simulink model "six_rod_tensegrity_model_2021a"  (R2021a)
settings: Solver=ode45  StartTime=0  StopTime=Inf  RelTol=1e-1
values from neighbouring files (symbols this model uses):
  grivity_z = -9.80665    [code_for_6_rods_tensegrity.m]
  i = 19    [drive_params.m]
  Jsum = Jd + Jp + Jnagr    (= 9.27e-08)    [drive_params.m]
  km = 9.32 / 1000    (= 0.00932)    [drive_params.m]
  kpdr = 0.81    [drive_params.m]
  kw = 60 / (2*pi * 1020)    (= 0.00936205547599)    [drive_params.m]
  L = 0.14 / 1000    (= 0.00014)    [drive_params.m]
  load_mass = 0.5    [code_for_6_rods_tensegrity.m]
  plane_offset = -(rod_length/2 + 0.032 + rod_radius)    [code_for_6_rods_tensegrity.m]
  R = 5.3    [drive_params.m]
  rod_end_drive_offset = spool_active_length    (= 0.015)    [code_for_6_rods_tensegrity.m]
  rod_end_mass = 0.05    [code_for_6_rods_tensegrity.m]
  rod_end_mass_with_drive = 0.2    [code_for_6_rods_tensegrity.m]
  rod_mass = 0.028    [code_for_6_rods_tensegrity.m]
  rod_mass_with_drive = 0.038    [code_for_6_rods_tensegrity.m]
  rod_radius = 0.004    [code_for_6_rods_tensegrity.m]
undefined symbols (not defined in the file or in its folder): Left_end_cap_1_1, Left_end_cap_2_3, Left_end_cap_3_5, Left_end_cap_4_7, Left_end_cap_5_9, Left_end_cap_6_11, Right_end_cap_1_2, Right_end_cap_2_4, Right_end_cap_3_6, Right_end_cap_4_8, Right_end_cap_5_10, Right_end_cap_6_12, Rod_center_1, Rod_center_2, Rod_center_3, Rod_center_4, Rod_center_5, Rod_center_6, sigbuilder_block, X, Y, Z
libraries: sm_lib x403, nesl_utility x73
(part 1 of 5)
settings Model: SimulationMode=accelerator  Creator=skept  LastModifiedBy=Alexander
settings SolverCC: ZeroCrossAlgorithm=Adaptive  AlgebraicLoopSolver=TrustRegion  MinimalZcImpactIntegration=on
settings DataIOCC: LimitDataPoints=on  ReturnWorkspaceOutputs=off
settings OptimizationCC: LifeSpan=Inf
settings DebuggingCC: ReadBeforeWriteMsg=DisableAll  WriteAfterWriteMsg=DisableAll  WriteAfterReadMsg=DisableAll  IgnoredZcDiagnostic=none  MultiTaskDSMMsg=none  SFMachineParentedDataDiag=warning  ArithmeticOperatorsInVariantConditions=warning
settings ModelReferenceCC: UpdateModelReferenceTargets=IfOutOfDate
settings SFSimCC: CustomCodeUndefinedFunction=UseInterfaceOnly  SimTargetLang=C++
settings ExplorerConfigSet: InternalSimMechanicsExplorerSettings="<ExplorerConfiguration><canonicalview>default</canonicalview><AnimationSetting><BasePlaybackSpeed>1.0</BasePlaybackSpeed><PlaybackSpeedFactor>1.0</PlaybackSpeedFactor></AnimationSetting><TilePanel><TileInfo><Tiles Columns=\"2\" Count=\"2\" Rows=\"1\"><Column Weight=\"0.4996\"/><Column Weight=\"0.5004\"/><Row Weight=\"1\"/><Tile Height=\"1\" Width=\"1\" X=\"0\" Y=\"0\"/><Tile Height=\"1\" Width=\"1\" X=\"1\" Y=\"0\"/></Tiles></TileInfo><SceneInfo><SceneViewer><BGColor><R>0.60000002384185791</R><G>0.60000002384185791</G><B>0.60000002384185791</B></BGColor><Camera><DoPerspective>off</DoPerspective><Position><X>4.6237270475932446</X><Y>-3.24046644242923998</Y><Z>4.39238714743132519</Z></Position><Center><X>-0.0432625823170843388</X><Y>0.165607191250739916</Y><Z>-0.253002280802875512</Z></Center><Up><X>-0.498867944911503491</X><Y>0.379278649695632186</Y><Z>0.779280744933962821</Z></Up><ViewLimDist>1</ViewLimDist><YLim>1.22665931905449344</YLim><XLim>0.999371665877494042</XLim></Camera></SceneViewer><SceneViewer><BGColor><R>0.60000002384185791</R><G>0.60000002384185791</G><B>0.60000002384185791</B></BGColor><Camera><DoPerspective>off</DoPerspective><Position><X>0.00285027965081703291</X><Y>-7.09077849007995908</Y><Z>0.0787782984999531449</Z></Position><Center><X>0.00285027965081703291</X><Y>1.92077906472493121e-07</Y><Z>0.0787782984999531449</Z></Center><Up><X>0</X><Y>-0</Y><Z>1</Z></Up><ViewLimDist>1</ViewLimDist><YLim>0.451172617625770545</YLim><XLim>0.368213013253280874</XLim></Camera></SceneViewer></SceneInfo></TilePanel><MechEditorPanel><Cameras/><GfxPanelCameraMap/><VideoCreator><PlaybackSpeedRatio>1.0</PlaybackSpeedRatio><FrameRate>60</FrameRate><VideoFormat>MPEG-4</VideoFormat><FrameSize>[1920 1080]</FrameSize></VideoCreator></MechEditorPanel></ExplorerConfiguration>"

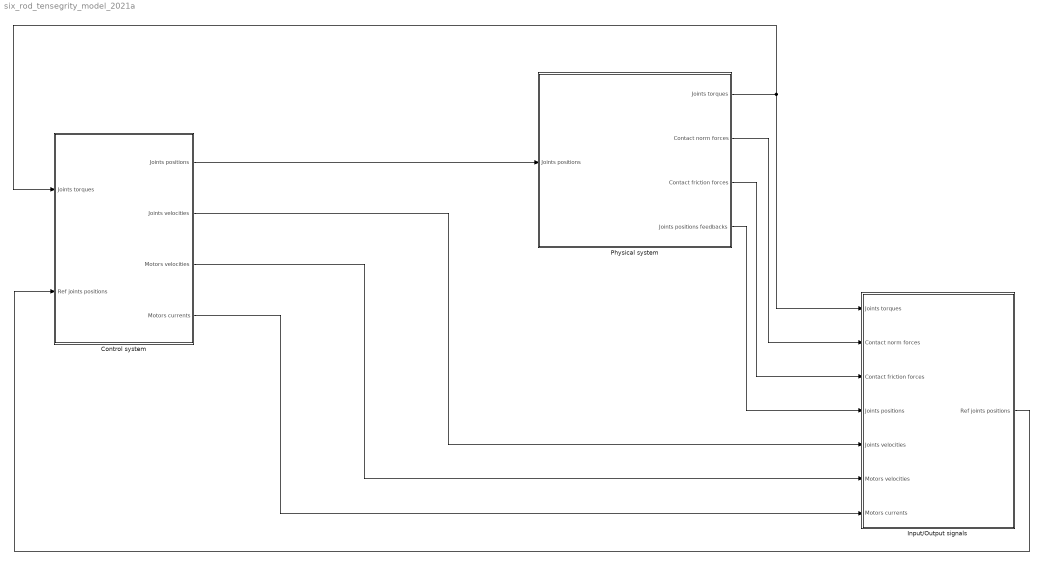
== system six_rod_tensegrity_model_2021a ==
  Control system : Subsystem
  Input/Output signals : Subsystem
  Physical system : Subsystem
      mask Display: image('$imagefile'); % Use "Edit Image" on toolstrip to change.
  wires:
  Control system/1(Joints positions) -> Physical system/1(Joints positions)
  Physical system/1(Joints torques) -> Input/Output signals/1(Joints torques), Control system/1(Joints torques)
  Control system/2(Joints velocities) -> Input/Output signals/5(Joints velocities)
  Control system/3(Motors velocities) -> Input/Output signals/6(Motors velocities)
  Control system/4(Motors currents) -> Input/Output signals/7(Motors currents)
  Input/Output signals/1(Ref joints positions) -> Control system/2(Ref joints positions)
  Physical system/2(Contact norm forces) -> Input/Output signals/2(Contact norm forces)
  Physical system/3(Contact friction forces) -> Input/Output signals/3(Contact friction forces)
  Physical system/4(Joints positions feedbacks) -> Input/Output signals/4(Joints positions)

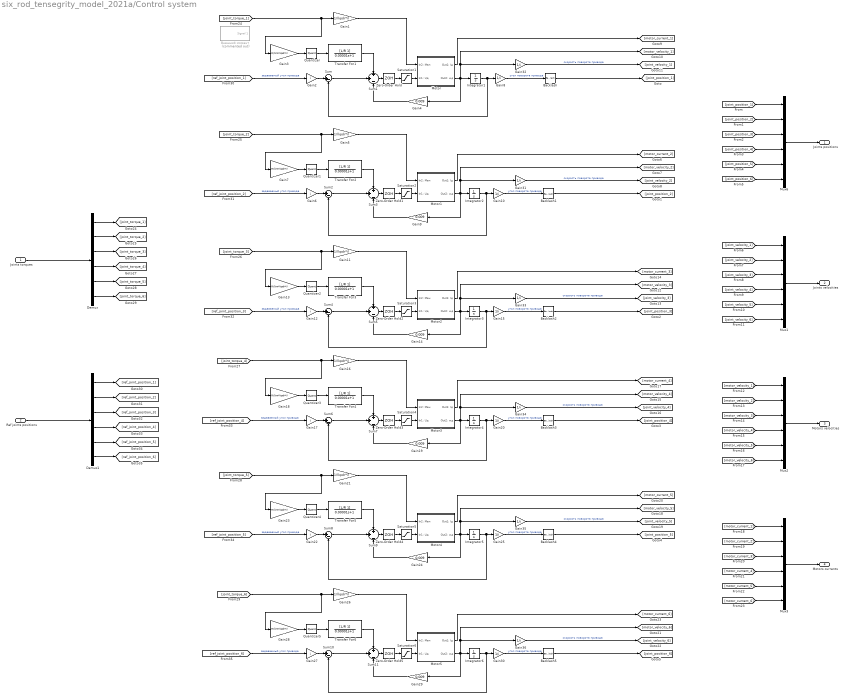
== system six_rod_tensegrity_model_2021a/Control system ==
  Joints torques : Inport
  Ref joints positions : Inport  Port=2
  Backlash{,1..5} (6 alike) : Backlash  BacklashWidth=0.0279
  Demux : Demux  Outputs=6
  Demux1 : Demux  Outputs=6
  Gain{1,5,11,16,21,26} (6 alike) : Gain  Gain=1/(kpdr*i)
  Gain{8,10,15,20,25,30..36} (12 alike) : Gain  Gain=1/i
  Gain{2,6,12,17,22,27} (6 alike) : Gain  Gain=i
  Gain{3,7,13,18,23,28} (6 alike) : Gain  Gain=R/(km*kpdr*i)
  Gain{4,9,14,19,24,29} (6 alike) : Gain  Gain=0.009
  Integrator{1..6} (6 alike) : Integrator
  Motor : Subsystem
  Motor1 : Subsystem
  Motor2 : Subsystem
  Motor3 : Subsystem
  Motor4 : Subsystem
  Motor5 : Subsystem
  Mux{1..3,6} (4 alike) : Mux  Inputs=6
  Quantizer{,1..5} (6 alike) : Quantizer  QuantizationInterval=0.00488
  Saturation{1..6} (6 alike) : Saturate  UpperLimit=10.8  LowerLimit=-10.8
  Sum{,2,4,6,8,10} (6 alike) : Sum  Inputs=|+-
  Sum{1,3,5,7,9,11} (6 alike) : Sum  Inputs=+|+|-
  Transfer Fcn{1..6} (6 alike) : TransferFcn  Numerator=[L/R 1]  Denominator=[0.00001 1]
  Zero-Order Hold{,1..5} (6 alike) : ZeroOrderHold  SampleTime=0.005
  Внешний момент : Subsystem  Tag=STV Subsys  Commented=on  LoadFcn=sigbuilder_block('load');  StartFcn=sigbuilder_block('start');  StopFcn=sigbuilder_block('stop');  ClipboardFcn=sigbuilder_block('clipboard');  mask(Sigbuilder block){tuvar=[0:10]}
      mask help: Simulink:masks:SigbuilderBlock_MD
      mask init:
      | if ~strcmp(get_param(bdroot(gcbh),'SimulationStatus'),'stopped') tuvar = sigbuilder_block('maskInit'); end
      settings: CopyFcn=sigbuilder_block('copy');  DeleteFcn=sigbuilder_block('delete');  ModelCloseFcn=sigbuilder_block('modelClose');  PreSaveFcn=sigbuilder_block('preSave');  PauseFcn=sigbuilder_block('pause');  ContinueFcn=sigbuilder_block('continue');  NameChangeFcn=sigbuilder_block('namechange');  OpenFcn=sigbuilder_block('open',[512.25 154.5 550.5 399.75 ]);  CloseFcn=sigbuilder_block('close');
      mask Display: plot(0, 0, 100, 100,[2, 2, 32, 32, 2], [68, 8, 8, 68, 68],[32, 2], [38, 38], [32, 19, 2],[53, 60, 44], [32, 17, 17, 2],[16, 16, 31, 31]);txt = getActiveGroup(gcbh);text(2, 100, txt,'verticalAlignment', 'top');
  Joints positions : Outport
  Joints velocities : Outport  Port=2
  Motors velocities : Outport  Port=3
  Motors currents : Outport  Port=4
  wires:
  Gain1/1 -> Motor/1(In2: Mвн)
  Backlash/1 -> [joint_position_1]
  [joint_torque_1] -> Gain1/1, Gain3/1
  Quantizer/1 -> Transfer Fcn1/1
  Gain4/1 -> Sum1/3
  Gain2/1 -> Sum/1
  Sum/1 -> Sum1/2
  Transfer Fcn1/1 -> Sum1/1
  Gain3/1 -> Quantizer/1
  [ref_joint_position_1] -> Gain2/1  "задаваемый угол привода"
  Integrator1/1 -> Gain8/1, Sum/2
  Zero-Order Hold/1 -> Saturation1/1
  Saturation1/1 -> Motor/2(In1: Uд)
  Sum1/1 -> Zero-Order Hold/1
  Motor/2(Out2: wд) -> [motor_velocity_1], Gain32/1, Integrator1/1, Gain4/1
  Gain8/1 -> Backlash/1  "угол поворота привода"
  Motor1/2(Out2: wд) -> Gain31/1, [motor_velocity_2], Gain9/1, Integrator2/1
  Integrator2/1 -> Gain10/1, Sum2/2
  Zero-Order Hold1/1 -> Saturation2/1
  Gain10/1 -> Backlash1/1  "угол поворота привода"
  Sum3/1 -> Zero-Order Hold1/1
  Transfer Fcn2/1 -> Sum3/1
  Gain9/1 -> Sum3/3
  [ref_joint_position_2] -> Gain6/1  "задаваемый угол привода"
  Gain7/1 -> Quantizer1/1
  Sum2/1 -> Sum3/2
  [joint_torque_2] -> Gain5/1, Gain7/1
  Quantizer1/1 -> Transfer Fcn2/1
  Gain6/1 -> Sum2/1
  Backlash1/1 -> [joint_position_2]
  Gain5/1 -> Motor1/1(In2: Mвн)
  Saturation2/1 -> Motor1/2(In1: Uд)
  Motor2/2(Out2: wд) -> Gain33/1, [motor_velocity_3], Gain14/1, Integrator3/1
  Integrator3/1 -> Gain15/1, Sum4/2
  Zero-Order Hold2/1 -> Saturation3/1
  Gain15/1 -> Backlash2/1  "угол поворота привода"
  Sum5/1 -> Zero-Order Hold2/1
  Transfer Fcn3/1 -> Sum5/1
  Gain14/1 -> Sum5/3
  [ref_joint_position_3] -> Gain12/1  "задаваемый угол привода"
  Gain13/1 -> Quantizer2/1
  Sum4/1 -> Sum5/2
  [joint_torque_3] -> Gain11/1, Gain13/1
  Quantizer2/1 -> Transfer Fcn3/1
  Gain12/1 -> Sum4/1
  Backlash2/1 -> [joint_position_3]
  Gain11/1 -> Motor2/1(In2: Mвн)
  Saturation3/1 -> Motor2/2(In1: Uд)
  Motor3/2(Out2: wд) -> [motor_velocity_4], Gain34/1, Integrator4/1, Gain19/1
  Integrator4/1 -> Gain20/1, Sum6/2
  Zero-Order Hold3/1 -> Saturation4/1
  Gain20/1 -> Backlash3/1  "угол поворота привода"
  Sum7/1 -> Zero-Order Hold3/1
  Transfer Fcn4/1 -> Sum7/1
  Gain19/1 -> Sum7/3
  [ref_joint_position_4] -> Gain17/1  "задаваемый угол привода"
  Gain18/1 -> Quantizer3/1
  Sum6/1 -> Sum7/2
  [joint_torque_4] -> Gain16/1, Gain18/1
  Quantizer3/1 -> Transfer Fcn4/1
  Gain17/1 -> Sum6/1
  Backlash3/1 -> [joint_position_4]
  Gain16/1 -> Motor3/1(In2: Mвн)
  Saturation4/1 -> Motor3/2(In1: Uд)
  Integrator5/1 -> Gain25/1, Sum8/2
  Zero-Order Hold4/1 -> Saturation5/1
  Gain25/1 -> Backlash4/1  "угол поворота привода"
  Sum9/1 -> Zero-Order Hold4/1
  Transfer Fcn5/1 -> Sum9/1
  Gain24/1 -> Sum9/3
  [ref_joint_position_5] -> Gain22/1  "задаваемый угол привода"
  Gain23/1 -> Quantizer4/1
  Sum8/1 -> Sum9/2
  [joint_torque_5] -> Gain21/1, Gain23/1
  Quantizer4/1 -> Transfer Fcn5/1
  Gain22/1 -> Sum8/1
  Backlash4/1 -> [joint_position_5]
  Gain21/1 -> Motor4/1(In2: Mвн)
  Saturation5/1 -> Motor4/2(In1: Uд)
  Motor5/2(Out2: wд) -> [motor_velocity_6], Gain36/1, Integrator6/1, Gain29/1
  Integrator6/1 -> Gain30/1, Sum10/2
  Zero-Order Hold5/1 -> Saturation6/1
  Gain30/1 -> Backlash5/1  "угол поворота привода"
  Sum11/1 -> Zero-Order Hold5/1
  Transfer Fcn6/1 -> Sum11/1
  Gain29/1 -> Sum11/3
  [ref_joint_position_6] -> Gain27/1  "задаваемый угол привода"
  Gain28/1 -> Quantizer5/1
  Sum10/1 -> Sum11/2
  [joint_torque_6] -> Gain26/1, Gain28/1
  Quantizer5/1 -> Transfer Fcn6/1
  Gain27/1 -> Sum10/1
  Backlash5/1 -> [joint_position_6]
  Gain26/1 -> Motor5/1(In2: Mвн)
  Saturation6/1 -> Motor5/2(In1: Uд)
  Mux6/1 -> Joints positions/1
  [joint_position_6] -> Mux6/6
  [joint_position_5] -> Mux6/5
  [joint_position_4] -> Mux6/4
  [joint_position_3] -> Mux6/3
  [joint_position_2] -> Mux6/2
  [joint_position_1] -> Mux6/1
  Motor1/1(Out1: Iд) -> [motor_current_2]
  Gain31/1 -> [joint_velocity_2]  "скорость поворота привода"
  Gain32/1 -> [joint_velocity_1]  "скорость поворота привода"
  Motor/1(Out1: Iд) -> [motor_current_1]
  Gain33/1 -> [joint_velocity_3]  "скорость поворота привода"
  Motor2/1(Out1: Iд) -> [motor_current_3]
  Gain34/1 -> [joint_velocity_4]  "скорость поворота привода"
  Motor3/1(Out1: Iд) -> [motor_current_4]
  Gain35/1 -> [joint_velocity_5]  "скорость поворота привода"
  Motor4/2(Out2: wд) -> Gain24/1, Gain35/1, [motor_velocity_5], Integrator5/1
  Motor4/1(Out1: Iд) -> [motor_current_5]
  Gain36/1 -> [joint_velocity_6]  "скорость поворота привода"
  Motor5/1(Out1: Iд) -> [motor_current_6]
  [joint_velocity_2] -> Mux1/2
  [joint_velocity_1] -> Mux1/1
  [joint_velocity_3] -> Mux1/3
  Mux1/1 -> Joints velocities/1
  [joint_velocity_4] -> Mux1/4
  [joint_velocity_5] -> Mux1/5
  [joint_velocity_6] -> Mux1/6
  [motor_velocity_2] -> Mux2/2
  [motor_velocity_1] -> Mux2/1
  [motor_velocity_3] -> Mux2/3
  Mux2/1 -> Motors velocities/1
  [motor_velocity_4] -> Mux2/4
  [motor_velocity_5] -> Mux2/5
  [motor_velocity_6] -> Mux2/6
  [motor_current_2] -> Mux3/2
  [motor_current_1] -> Mux3/1
  [motor_current_3] -> Mux3/3
  Mux3/1 -> Motors currents/1
  [motor_current_4] -> Mux3/4
  [motor_current_5] -> Mux3/5
  [motor_current_6] -> Mux3/6
  Demux/1 -> [joint_torque_1]
  Demux/2 -> [joint_torque_2]
  Demux/3 -> [joint_torque_3]
  Demux/6 -> [joint_torque_6]
  Joints torques/1 -> Demux/1
  Demux/4 -> [joint_torque_4]
  Demux/5 -> [joint_torque_5]
  Demux1/6 -> [ref_joint_position_6]
  Demux1/3 -> [ref_joint_position_3]
  Demux1/1 -> [ref_joint_position_1]
  Demux1/2 -> [ref_joint_position_2]
  Ref joints positions/1 -> Demux1/1
  Demux1/4 -> [ref_joint_position_4]
  Demux1/5 -> [ref_joint_position_5]

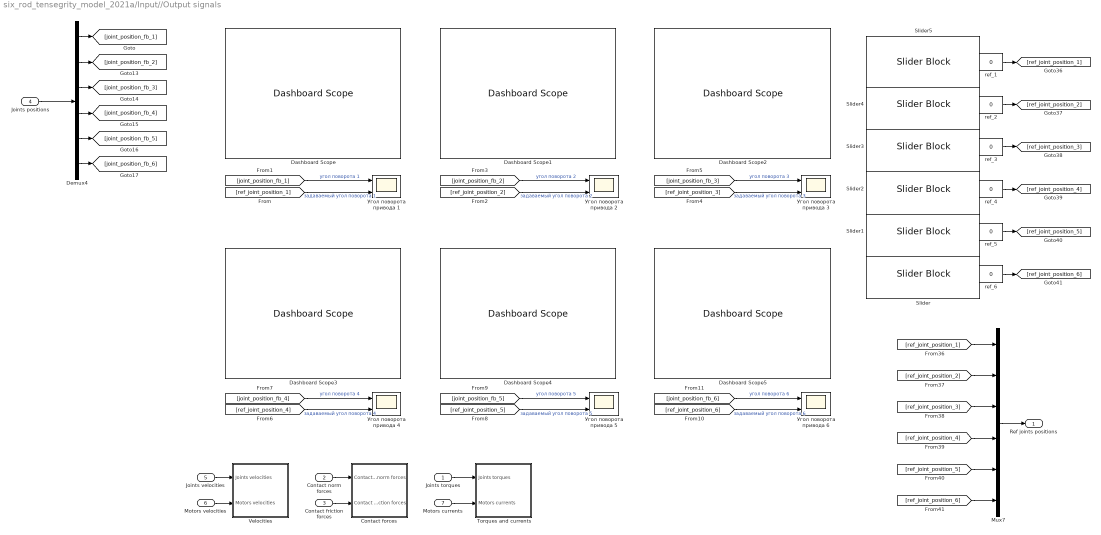
== system six_rod_tensegrity_model_2021a/Input//Output signals ==
  Joints torques : Inport
  Contact norm forces : Inport  Port=2
  Contact friction forces : Inport  Port=3
  Joints positions : Inport  Port=4
  Joints velocities : Inport  Port=5
  Motors velocities : Inport  Port=6
  Motors currents : Inport  Port=7
  Contact forces : Subsystem
  Dashboard Scope{,1..5} (6 alike) : DashboardScope
  Demux4 : Demux  Outputs=6
  Mux7 : Mux  Inputs=6
  Slider{,1..5} (6 alike) : SliderBlock  ScaleMax=200
  Torques and currents : Subsystem
  Velocities : Subsystem
  ref_{1..6} (6 alike) : Constant  Value=0
  Угол поворота привода {1..6} (6 alike) : Scope  NumInputPorts=2
  Ref joints positions : Outport
  wires:
  Demux4/1 -> [joint_position_fb_1]
  Demux4/2 -> [joint_position_fb_2]
  Demux4/3 -> [joint_position_fb_3]
  Demux4/6 -> [joint_position_fb_6]
  Joints positions/1 -> Demux4/1
  Demux4/4 -> [joint_position_fb_4]
  Demux4/5 -> [joint_position_fb_5]
  [ref_joint_position_1] -> Угол поворота привода 1/2  "задаваемый угол поворота 1"
  [joint_position_fb_1] -> Угол поворота привода 1/1  "угол поворота 1"
  [joint_position_fb_2] -> Угол поворота привода 2/1  "угол поворота 2"
  [ref_joint_position_2] -> Угол поворота привода 2/2  "задаваемый угол поворота 2"
  [joint_position_fb_3] -> Угол поворота привода 3/1  "угол поворота 3"
  [ref_joint_position_3] -> Угол поворота привода 3/2  "задаваемый угол поворота 3"
  [joint_position_fb_4] -> Угол поворота привода 4/1  "угол поворота 4"
  [ref_joint_position_4] -> Угол поворота привода 4/2  "задаваемый угол поворота 4"
  [joint_position_fb_5] -> Угол поворота привода 5/1  "угол поворота 5"
  [ref_joint_position_5] -> Угол поворота привода 5/2  "задаваемый угол поворота 5"
  [joint_position_fb_6] -> Угол поворота привода 6/1  "угол поворота 6"
  [ref_joint_position_6] -> Угол поворота привода 6/2  "задаваемый угол поворота 6"
  ref_5/1 -> [ref_joint_position_5]
  ref_2/1 -> [ref_joint_position_2]
  ref_6/1 -> [ref_joint_position_6]
  ref_4/1 -> [ref_joint_position_4]
  ref_1/1 -> [ref_joint_position_1]
  [ref_joint_position_1] -> Mux7/1
  [ref_joint_position_5] -> Mux7/5
  Mux7/1 -> Ref joints positions/1
  [ref_joint_position_3] -> Mux7/3
  [ref_joint_position_6] -> Mux7/6
  [ref_joint_position_4] -> Mux7/4
  [ref_joint_position_2] -> Mux7/2
  ref_3/1 -> [ref_joint_position_3]
  Contact norm forces/1 -> Contact forces/1(Contact norm forces)
  Contact friction forces/1 -> Contact forces/2(Contact friction forces)
  Joints velocities/1 -> Velocities/1(Joints velocities)
  Motors velocities/1 -> Velocities/2(Motors velocities)
  Joints torques/1 -> Torques and currents/1(Joints torques)
  Motors currents/1 -> Torques and currents/2(Motors currents)

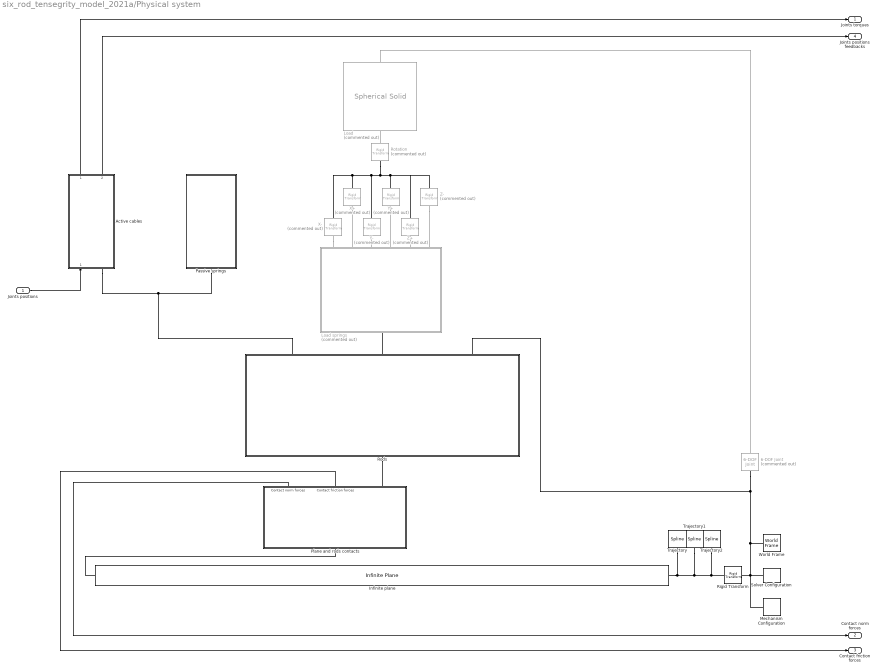
== system six_rod_tensegrity_model_2021a/Physical system ==
  Joints positions : Inport
  6-DOF Joint : sm_lib/Joints/6-DOF Joint  Commented=on  JointMode=Normal  SenseConstraintForce=off  SenseConstraintForceX=off  SenseConstraintForceY=off  SenseConstraintForceZ=off  SenseConstraintTorque=off  SenseConstraintTorqueX=off  SenseConstraintTorqueY=off  SenseConstraintTorqueZ=off  SenseTotalForce=off  SenseTotalForceX=off  SenseTotalForceY=off  SenseTotalForceZ=off  SenseTotalTorque=off  SenseTotalTorqueX=off  SenseTotalTorqueY=off  SenseTotalTorqueZ=off  CompositeWrenchDir=FollowerOnBase  CompositeWrenchFrame=BaseFrame  PxEquilibriumPosition=0  PxEquilibriumPositionUnits=m  PxSpringStiffness=0  PxSpringStiffnessUnits=N/m  PxDampingCoefficient=0  PxDampingCoefficientUnits=N/(m/s)  PxTorqueActuationMode=NoTorque  PxMotionActuationMode=ComputedMotion  PxSensePosition=off  PxSenseVelocity=off  PxSenseAcceleration=off  PxSenseTorqueForce=off  PxSenseLowerLimitTorqueForce=off  PxSenseUpperLimitTorqueForce=off  PxLowerLimitSpecify=off  PxLowerLimitBound=-1  PxLowerLimitBoundUnits=m  PxLowerLimitStiffness=1e6  PxLowerLimitStiffnessUnits=N/m  PxLowerLimitDamping=1e3  PxLowerLimitDampingUnits=N/(m/s)  PxLowerLimitTransitionRegionWidth=1e-4  PxLowerLimitTransitionRegionWidthUnits=m  PxUpperLimitSpecify=off  PxUpperLimitBound=1  PxUpperLimitBoundUnits=m  PxUpperLimitStiffness=1e6  PxUpperLimitStiffnessUnits=N/m  PxUpperLimitDamping=1e3  PxUpperLimitDampingUnits=N/(m/s)  PxUpperLimitTransitionRegionWidth=1e-4  PxUpperLimitTransitionRegionWidthUnits=m  PxPositionTargetSpecify=off  PxPositionTargetPriority=High  PxPositionTargetValue=0  PxPositionTargetValueUnits=m  PxVelocityTargetSpecify=off  PxVelocityTargetPriority=High  PxVelocityTargetValue=0  PxVelocityTargetValueUnits=m/s  PyEquilibriumPosition=0  PyEquilibriumPositionUnits=m  PySpringStiffness=0  PySpringStiffnessUnits=N/m  PyDampingCoefficient=0  PyDampingCoefficientUnits=N/(m/s)  PyTorqueActuationMode=NoTorque  PyMotionActuationMode=ComputedMotion  PySensePosition=off  PySenseVelocity=off  PySenseAcceleration=off  PySenseTorqueForce=off  PySenseLowerLimitTorqueForce=off  PySenseUpperLimitTorqueForce=off  PyLowerLimitSpecify=off  PyLowerLimitBound=-1  PyLowerLimitBoundUnits=m  PyLowerLimitStiffness=1e6  PyLowerLimitStiffnessUnits=N/m  PyLowerLimitDamping=1e3  PyLowerLimitDampingUnits=N/(m/s)  PyLowerLimitTransitionRegionWidth=1e-4  PyLowerLimitTransitionRegionWidthUnits=m  PyUpperLimitSpecify=off  PyUpperLimitBound=1  PyUpperLimitBoundUnits=m  PyUpperLimitStiffness=1e6  PyUpperLimitStiffnessUnits=N/m  PyUpperLimitDamping=1e3  PyUpperLimitDampingUnits=N/(m/s)  PyUpperLimitTransitionRegionWidth=1e-4  PyUpperLimitTransitionRegionWidthUnits=m  PyPositionTargetSpecify=off  PyPositionTargetPriority=High  PyPositionTargetValue=0  PyPositionTargetValueUnits=m  PyVelocityTargetSpecify=off  PyVelocityTargetPriority=High  PyVelocityTargetValue=0  PyVelocityTargetValueUnits=m/s  PzEquilibriumPosition=0  PzEquilibriumPositionUnits=m  PzSpringStiffness=0  PzSpringStiffnessUnits=N/m  PzDampingCoefficient=0  PzDampingCoefficientUnits=N/(m/s)  PzTorqueActuationMode=NoTorque  PzMotionActuationMode=ComputedMotion  PzSensePosition=off  PzSenseVelocity=off  PzSenseAcceleration=off  PzSenseTorqueForce=off  PzSenseLowerLimitTorqueForce=off  PzSenseUpperLimitTorqueForce=off  PzLowerLimitSpecify=off  PzLowerLimitBound=-1  PzLowerLimitBoundUnits=m  PzLowerLimitStiffness=1e6  PzLowerLimitStiffnessUnits=N/m  PzLowerLimitDamping=1e3  PzLowerLimitDampingUnits=N/(m/s)  PzLowerLimitTransitionRegionWidth=1e-4  PzLowerLimitTransitionRegionWidthUnits=m  PzUpperLimitSpecify=off  PzUpperLimitBound=1  PzUpperLimitBoundUnits=m  PzUpperLimitStiffness=1e6  PzUpperLimitStiffnessUnits=N/m  PzUpperLimitDamping=1e3  PzUpperLimitDampingUnits=N/(m/s)  PzUpperLimitTransitionRegionWidth=1e-4  PzUpperLimitTransitionRegionWidthUnits=m  PzPositionTargetSpecify=off  PzPositionTargetPriority=High  PzPositionTargetValue=0  PzPositionTargetValueUnits=m  PzVelocityTargetSpecify=off  PzVelocityTargetPriority=High  PzVelocityTargetValue=0  PzVelocityTargetValueUnits=m/s  SphDefPosRotationMethod=None  SphDefPosRotationAngleUnits=deg  SphDefPosRotationStandardAxis=+Z  SphDefPosRotationAngle=0.0  SphDefPosRotationArbitraryAxis=[0 0 1]  SphDefPosFollAlignAxisA=+X  SphDefPosBaseAlignAxisA=+Y  SphDefPosFollAlignAxisB=+Y  SphDefPosBaseAlignAxisB=+Z  SphDefPosRotationSequenceAxes=FollowerAxes  SphDefPosRotationSequence=XYX  SphDefPosRotationSequenceAngles=[0 0 0]  SphDefPosRotationSequenceAnglesUnits=deg  SphDefPosRotationMatrix=[1 0 0; 0 1 0; 0 0 1]  SphEqPosRotationMethod=None  SphEqPosRotationAngleUnits=deg  SphEqPosRotationStandardAxis=+Z  SphEqPosRotationAngle=0.0  SphEqPosRotationArbitraryAxis=[0 0 1]  SphEqPosFollAlignAxisA=+X  SphEqPosBaseAlignAxisA=+Y  SphEqPosFollAlignAxisB=+Y  SphEqPosBaseAlignAxisB=+Z  SphEqPosRotationSequenceAxes=FollowerAxes  SphEqPosRotationSequence=XYX  SphEqPosRotationSequenceAngles=[0 0 0]  SphEqPosRotationSequenceAnglesUnits=deg  SphEqPosRotationMatrix=[1 0 0; 0 1 0; 0 0 1]  SphSpringStiffness=0  SphSpringStiffnessUnits=N*m/deg  SphDampingCoefficient=0  SphDampingCoefficientUnits=N*m/(deg/s)  SphActuateTorqueX=off  SphActuateTorqueY=off  SphActuateTorqueZ=off  SphActuateTorque=off  SphTorqueActuationMode=NoTorque  SphMotionActuationMode=ComputedMotion  SphActuationFrame=BaseFrame  SphSensePosition=off  SphSenseVelocityX=off  SphSenseVelocityY=off  SphSenseVelocityZ=off  SphSenseVelocity=off  SphSenseAccelerationX=off  SphSenseAccelerationY=off  SphSenseAccelerationZ=off  SphSenseAcceleration=off  SphSenseTorqueX=off  SphSenseTorqueY=off  SphSenseTorqueZ=off  SphSenseTorqueForce=off  SphSenseLowerLimitTorqueMag=off  SphSenseUpperLimitTorqueMag=off  SphSensingFrame=BaseFrame  SphLowerLimitSpecify=off  SphLowerLimitBound=15  SphLowerLimitBoundUnits=deg  SphLowerLimitStiffness=1e4  SphLowerLimitStiffnessUnits=N*m/deg  SphLowerLimitDamping=10  SphLowerLimitDampingUnits=N*m/(deg/s)  SphLowerLimitTransitionRegionWidth=0.1  SphLowerLimitTransitionRegionWidthUnits=deg  SphUpperLimitSpecify=off  SphUpperLimitBound=45  SphUpperLimitBoundUnits=deg  SphUpperLimitStiffness=1e4  SphUpperLimitStiffnessUnits=N*m/deg  SphUpperLimitDamping=10  SphUpperLimitDampingUnits=N*m/(deg/s)  SphUpperLimitTransitionRegionWidth=0.1  SphUpperLimitTransitionRegionWidthUnits=deg  SphPositionTargetRotationMethod=None  SphPositionTargetRotationAngleUnits=deg  SphPositionTargetRotationStandardAxis=+Z  SphPositionTargetRotationAngle=0.0  SphPositionTargetRotationArbitraryAxis=[0 0 1]  SphPositionTargetFollAlignAxisA=+X  SphPositionTargetBaseAlignAxisA=+Y  SphPositionTargetFollAlignAxisB=+Y  SphPositionTargetBaseAlignAxisB=+Z  SphPositionTargetRotationSequenceAxes=FollowerAxes  SphPositionTargetRotationSequence=XYX  SphPositionTargetRotationSequenceAngles=[0 0 0]  SphPositionTargetRotationSequenceAnglesUnits=deg  SphPositionTargetRotationMatrix=[1 0 0; 0 1 0; 0 0 1]  SphPositionTargetSpecify=off  SphPositionTargetPriority=High  SphVelocityTargetValue=[0 0 0]  SphVelocityTargetValueUnits=deg/s  SphVelocityTargetSpecify=off  SphVelocityTargetPriority=High  SphVelocityTargetInFollowerFrame=on
  Active cables : Subsystem
  Infinite plane : sm_lib/Curves and Surfaces/Infinite Plane  GraphicType=Rectangle  GraphicPlaneWidth=plane_length_x  GraphicPlaneWidthUnits=m  GraphicPlaneHeight=plane_length_y  GraphicPlaneHeightUnits=m  GraphicVisPropType=SimpleVisualProperties  GraphicDiffuseColor=[0.502 0.502 0.502]  GraphicOpacity=0.25  GraphicSpecularColor=[0.5 0.1 0.75 1.0]  GraphicAmbientColor=[0.15 0.15 0.75 1.0]  GraphicEmissiveColor=[0.0 0.0 0.0 1.0]  GraphicShininess=100
  Load : sm_lib/Body Elements/Spherical Solid  Commented=on  GraphicAmbientColor=[0.15 0.15 0.15 1.0]  BasedOnType=Mass  CenterOfMass=[0 0 0]  CenterOfMassUnits=m  GraphicDiffuseColor=load_color  Density=1000  DensityUnits=kg/m^3  DoExposeReferenceFrame=on  GraphicEmissiveColor=[0.0 0.0 0.0 1.0]  ExportEntireGeometry=off  SerializedExposedGeometries=<ExposedGeometries/>  SerializedFrames=<Frames><Frame><Id>Frame1</Id><Value><Name>Springs</Name><Origin><Source>ReferenceFrame</Source><FeatureName></FeatureName></Origin><PrimaryAxis><DefinedDirection>+Z</DefinedDirection><Source>ReferenceFrame</Source><SourceDirection>+Z</SourceDirection><FeatureName></FeatureName></PrimaryAxis><SecondaryAxis><DefinedDirection>+X</DefinedDirection><Source>ReferenceFrame</Source><SourceDirection>+X</SourceDirection><FeatureName></FeatureName></SecondaryAxis></Value></Frame></Frames>  MarkerShape=Sphere  MarkerSize=10  GraphicType=FromGeometry  InertiaType=PointMass  Mass=load_mass  MassUnits=kg  MomentsOfInertia=[1 1 1]  MomentsOfInertiaUnits=kg*m^2  GraphicOpacity=load_opacity  ProductsOfInertia=[0 0 0]  ProductsOfInertiaUnits=kg*m^2  GraphicShininess=75  GraphicSpecularColor=[0.5 0.5 0.5 1.0]  SphereRadius=load_radius  SphereRadiusUnits=m  GraphicVisPropType=SimpleVisualProperties
  Load springs : Subsystem  Commented=on
  Mechanism Configuration : sm_lib/Utilities/Mechanism Configuration  UniformGravity=Constant  GravityVector=[0 0 grivity_z]  GravityVectorUnits=m/s^2  GravityUnits=m/s^2  LinearizationDelta=0.001  JointModeTransitionNonlinearIterations=2
  Passive springs : Subsystem
  Plane and rods contacts : Subsystem
      mask Display: image('$imagefile'); % Use "Edit Image" on toolstrip to change.
  Rigid Transform : sm_lib/Frames and Transforms/Rigid Transform  TranslationMethod=Cartesian  TranslationStandardOffset=100  TranslationLengthUnit=m  TranslationStandardAxis=-Z  TranslationCartesianOffset=[0 0 plane_offset]  TranslationROffset=0  TranslationROffsetUnits=m  TranslationZOffset=0  TranslationZOffsetUnits=m  TranslationThetaOffset=0  TranslationThetaOffsetUnits=deg  RotationMethod=None  RotationAngleUnits=deg  RotationStandardAxis=+Z  RotationAngle=0.0  RotationArbitraryAxis=[0 0 1]  FollAlignAxisA=+X  BaseAlignAxisA=+Y  FollAlignAxisB=+Y  BaseAlignAxisB=+Z  RotationSequenceAxes=FollowerAxes  RotationSequence=XYX  RotationSequenceAngles=[0 0 0]  RotationSequenceAnglesUnits=deg  RotationMatrix=[1 0 0; 0 1 0; 0 0 1]
  Rods : Subsystem
      mask Display: image('$imagefile'); % Use "Edit Image" on toolstrip to change.
  Rotation : sm_lib/Frames and Transforms/Rigid Transform  Commented=on  TranslationMethod=None  TranslationStandardOffset=load_radius  TranslationLengthUnit=m  TranslationStandardAxis=+X  TranslationCartesianOffset=[0 0 0]  TranslationROffset=0  TranslationROffsetUnits=m  TranslationZOffset=0  TranslationZOffsetUnits=m  TranslationThetaOffset=0  TranslationThetaOffsetUnits=deg  RotationMethod=RotationMatrix  RotationAngleUnits=deg  RotationStandardAxis=+Z  RotationAngle=0.0  RotationArbitraryAxis=[0 0 1]  FollAlignAxisA=+X  BaseAlignAxisA=+Y  FollAlignAxisB=+Y  BaseAlignAxisB=+Z  RotationSequenceAxes=FollowerAxes  RotationSequence=XYX  RotationSequenceAngles=[0 0 0]  RotationSequenceAnglesUnits=deg  RotationMatrix=rotation_matrix
  Solver Configuration : nesl_utility/Solver Configuration  PhysicalDomain=network_engine_domain  SubClassName=solver  LeftPortType=input  RightPortType=generic  Tones=[]  Harmonics=[]  SimulateNoise=off  Profile=off  UseLocalSampling=off  EnableSwitchedLinearOptims=on  FrequencyDomain=off  UseCCode=off  RelTol=0.001  AbsTol=1e-06  MinStep=1e-09  ToWorkspace=off  RevertToSquareIcSolve=off  NumHomotopyIterations=100  PhasorMode=off  PhasorModeNumHarmonics=1  DoDC=off  ResidualTolerance=1e-5  UseLocalSolver=off  LocalSolverChoice=NE_BACKWARD_EULER_ADVANCER  LocalSolverSampleTime=0.001  DoFixedCost=off  MaxNonlinIter=3  MaxModeIter=2  ComputeImpulses=off  ImpulseIterations=2  LinearAlgebra=Sparse  EquationFormulation=NE_TIME_EF  DelaysMemoryBudget=1024  AutomaticFiltering=on  FilteringTimeConstant=0.001  PartitionStorageMethod=AS_NEEDED  PartitionMemoryBudget=1024  PartitionMethod=FAST
      settings: SourceProductBaseCode=PW,SS
  Trajectory : sm_lib/Curves and Surfaces/Spline  GraphicAmbientColor=[0.15 0.15 0.15 1.0]  GraphicDiffuseColor=[0.0 0.0 0.0]  DataPoints=[0 0 0; 1 0 0; 2 0 0; 3 0 0; ]  DataPointsUnits=m  GraphicEmissiveColor=[0.0 0.0 0.0 1.0]  EndConditionType=Natural  MarkerShape=Sphere  MarkerSize=10  GraphicType=FromGeometry  GraphicOpacity=1.0  GraphicShininess=75  GraphicSpecularColor=[0.5 0.5 0.5 1.0]  GraphicVisPropType=SimpleVisualProperties
  Trajectory1 : sm_lib/Curves and Surfaces/Spline  GraphicAmbientColor=[0.15 0.15 0.15 1.0]  GraphicDiffuseColor=[0.0 0.0 0.0]  DataPoints=[1 0 0; 0 1 0; -1 0 0; 0 -1 0; 1 0 0;]  DataPointsUnits=m  GraphicEmissiveColor=[0.0 0.0 0.0 1.0]  EndConditionType=Natural  MarkerShape=Sphere  MarkerSize=10  GraphicType=FromGeometry  GraphicOpacity=1.0  GraphicShininess=75  GraphicSpecularColor=[0.5 0.5 0.5 1.0]  GraphicVisPropType=SimpleVisualProperties
  Trajectory2 : sm_lib/Curves and Surfaces/Spline  GraphicAmbientColor=[0.15 0.15 0.15 1.0]  GraphicDiffuseColor=[0.0 0.0 0.0]  DataPoints=[2 0 0; 0 2 0; -2 0 0; 0 -2 0; 2 0 0;]  DataPointsUnits=m  GraphicEmissiveColor=[0.0 0.0 0.0 1.0]  EndConditionType=Natural  MarkerShape=Sphere  MarkerSize=10  GraphicType=FromGeometry  GraphicOpacity=1.0  GraphicShininess=75  GraphicSpecularColor=[0.5 0.5 0.5 1.0]  GraphicVisPropType=SimpleVisualProperties
  World Frame : sm_lib/Frames and Transforms/World Frame
  X+ : sm_lib/Frames and Transforms/Rigid Transform  Commented=on  TranslationMethod=StandardAxis  TranslationStandardOffset=load_radius  TranslationLengthUnit=m  TranslationStandardAxis=+X  TranslationCartesianOffset=[0 0 0]  TranslationROffset=0  TranslationROffsetUnits=m  TranslationZOffset=0  TranslationZOffsetUnits=m  TranslationThetaOffset=0  TranslationThetaOffsetUnits=deg  RotationMethod=None  RotationAngleUnits=deg  RotationStandardAxis=+Z  RotationAngle=0.0  RotationArbitraryAxis=[0 0 1]  FollAlignAxisA=+X  BaseAlignAxisA=+Y  FollAlignAxisB=+Y  BaseAlignAxisB=+Z  RotationSequenceAxes=FollowerAxes  RotationSequence=XYX  RotationSequenceAngles=[0 0 0]  RotationSequenceAnglesUnits=deg  RotationMatrix=rotation_matrix
  X- : sm_lib/Frames and Transforms/Rigid Transform  Commented=on  TranslationMethod=StandardAxis  TranslationStandardOffset=load_radius  TranslationLengthUnit=m  TranslationStandardAxis=-X  TranslationCartesianOffset=[0 0 0]  TranslationROffset=0  TranslationROffsetUnits=m  TranslationZOffset=0  TranslationZOffsetUnits=m  TranslationThetaOffset=0  TranslationThetaOffsetUnits=deg  RotationMethod=None  RotationAngleUnits=deg  RotationStandardAxis=+Z  RotationAngle=0.0  RotationArbitraryAxis=[0 0 1]  FollAlignAxisA=+X  BaseAlignAxisA=+Y  FollAlignAxisB=+Y  BaseAlignAxisB=+Z  RotationSequenceAxes=FollowerAxes  RotationSequence=XYX  RotationSequenceAngles=[0 0 0]  RotationSequenceAnglesUnits=deg  RotationMatrix=rotation_matrix
  Y+ : sm_lib/Frames and Transforms/Rigid Transform  Commented=on  TranslationMethod=StandardAxis  TranslationStandardOffset=load_radius  TranslationLengthUnit=m  TranslationStandardAxis=+Y  TranslationCartesianOffset=[0 0 0]  TranslationROffset=0  TranslationROffsetUnits=m  TranslationZOffset=0  TranslationZOffsetUnits=m  TranslationThetaOffset=0  TranslationThetaOffsetUnits=deg  RotationMethod=None  RotationAngleUnits=deg  RotationStandardAxis=+Z  RotationAngle=0.0  RotationArbitraryAxis=[0 0 1]  FollAlignAxisA=+X  BaseAlignAxisA=+Y  FollAlignAxisB=+Y  BaseAlignAxisB=+Z  RotationSequenceAxes=FollowerAxes  RotationSequence=XYX  RotationSequenceAngles=[0 0 0]  RotationSequenceAnglesUnits=deg  RotationMatrix=rotation_matrix
  Y- : sm_lib/Frames and Transforms/Rigid Transform  Commented=on  TranslationMethod=StandardAxis  TranslationStandardOffset=load_radius  TranslationLengthUnit=m  TranslationStandardAxis=-Y  TranslationCartesianOffset=[0 0 0]  TranslationROffset=0  TranslationROffsetUnits=m  TranslationZOffset=0  TranslationZOffsetUnits=m  TranslationThetaOffset=0  TranslationThetaOffsetUnits=deg  RotationMethod=None  RotationAngleUnits=deg  RotationStandardAxis=+Z  RotationAngle=0.0  RotationArbitraryAxis=[0 0 1]  FollAlignAxisA=+X  BaseAlignAxisA=+Y  FollAlignAxisB=+Y  BaseAlignAxisB=+Z  RotationSequenceAxes=FollowerAxes  RotationSequence=XYX  RotationSequenceAngles=[0 0 0]  RotationSequenceAnglesUnits=deg  RotationMatrix=rotation_matrix
  Z+ : sm_lib/Frames and Transforms/Rigid Transform  Commented=on  TranslationMethod=StandardAxis  TranslationStandardOffset=load_radius  TranslationLengthUnit=m  TranslationStandardAxis=+Z  TranslationCartesianOffset=[0 0 0]  TranslationROffset=0  TranslationROffsetUnits=m  TranslationZOffset=0  TranslationZOffsetUnits=m  TranslationThetaOffset=0  TranslationThetaOffsetUnits=deg  RotationMethod=None  RotationAngleUnits=deg  RotationStandardAxis=+Z  RotationAngle=0.0  RotationArbitraryAxis=[0 0 1]  FollAlignAxisA=+X  BaseAlignAxisA=+Y  FollAlignAxisB=+Y  BaseAlignAxisB=+Z  RotationSequenceAxes=FollowerAxes  RotationSequence=XYX  RotationSequenceAngles=[0 0 0]  RotationSequenceAnglesUnits=deg  RotationMatrix=rotation_matrix
  Z- : sm_lib/Frames and Transforms/Rigid Transform  Commented=on  TranslationMethod=StandardAxis  TranslationStandardOffset=load_radius  TranslationLengthUnit=m  TranslationStandardAxis=-Z  TranslationCartesianOffset=[0 0 0]  TranslationROffset=0  TranslationROffsetUnits=m  TranslationZOffset=0  TranslationZOffsetUnits=m  TranslationThetaOffset=0  TranslationThetaOffsetUnits=deg  RotationMethod=None  RotationAngleUnits=deg  RotationStandardAxis=+Z  RotationAngle=0.0  RotationArbitraryAxis=[0 0 1]  FollAlignAxisA=+X  BaseAlignAxisA=+Y  FollAlignAxisB=+Y  BaseAlignAxisB=+Z  RotationSequenceAxes=FollowerAxes  RotationSequence=XYX  RotationSequenceAngles=[0 0 0]  RotationSequenceAnglesUnits=deg  RotationMatrix=rotation_matrix
  Joints torques : Outport
  Contact norm forces : Outport  Port=2
  Contact friction forces : Outport  Port=3
  Joints positions feedbacks : Outport  Port=4
  wires:
  Joints positions/1 -> Active cables/1(Joints positions)
  Active cables/1(Joints torques) -> Joints torques/1
  Plane and rods contacts/2(Contact friction forces) -> Contact friction forces/1
  Plane and rods contacts/1(Contact norm forces) -> Contact norm forces/1
  Active cables/2(Joints positions feedbacks) -> Joints positions feedbacks/1
  connections:
  Load/RConn1 -- 6-DOF Joint/RConn1
  Z+/RConn1 -- Load springs/RConn5
  Rods/RConn1 -- Plane and rods contacts/RConn1
  Y-/RConn1 -- Load springs/RConn3
  Y+/RConn1 -- Load springs/RConn4
  X+/RConn1 -- Load springs/RConn2
  X-/RConn1 -- Load springs/RConn1
  Z-/LConn1 -- Z+/LConn1 -- Rotation/RConn1 -- Y-/LConn1 -- X-/LConn1 -- X+/LConn1 -- Y+/LConn1
  Passive springs/LConn1 -- Active cables/LConn1 -- Rods/LConn1
  Infinite plane/LConn1 -- Trajectory/LConn1 -- Trajectory1/LConn1 -- Trajectory2/LConn1 -- Rigid Transform/RConn1
  Z-/RConn1 -- Load springs/RConn6
  Infinite plane/RConn1 -- Plane and rods contacts/LConn1
  Rods/LConn2 -- Load springs/LConn1
  Rods/LConn3 -- 6-DOF Joint/LConn1 -- World Frame/RConn1 -- Rigid Transform/LConn1 -- Mechanism Configuration/RConn1 -- Solver Configuration/RConn1
  Rotation/LConn1 -- Load/LConn1

== system six_rod_tensegrity_model_2021a/Control system/Motor ==
  In2: Mвн : Inport
  In1: Uд : Inport  Port=2
  Gain : Gain  Gain=km
  Gain1 : Gain  Gain=1/Jsum
  Gain2 : Gain  Gain=kw
  Integrator : Integrator
  Saturation1 : Saturate  UpperLimit=1.72  LowerLimit=-1.72
  Sum : Sum  Inputs=|+-
  Sum1 : Sum  Inputs=-+|
  Transfer Fcn : TransferFcn  Numerator=[1/R]  Denominator=[L/R 1]
  Out1: Iд : Outport  VectorParamsAs1DForOutWhenUnconnected=off
  Out2: wд : Outport  Port=2  VectorParamsAs1DForOutWhenUnconnected=off
  wires:
  In1: Uд/1 -> Sum/1
  Transfer Fcn/1 -> Saturation1/1  "Iд"
  Sum/1 -> Transfer Fcn/1  "Uд - E"
  Integrator/1 -> Out2: wд/1, Gain2/1  "скорость"
  Gain2/1 -> Sum/2  "E"
  Gain1/1 -> Integrator/1  "ускорение"
  Gain/1 -> Sum1/2  "Mд"
  In2: Mвн/1 -> Sum1/1
  Sum1/1 -> Gain1/1
  Saturation1/1 -> Out1: Iд/1, Gain/1

== system six_rod_tensegrity_model_2021a/Control system/Motor1 ==
  In2: Mвн : Inport
  In1: Uд : Inport  Port=2
  Gain : Gain  Gain=km
  Gain1 : Gain  Gain=1/Jsum
  Gain2 : Gain  Gain=kw
  Integrator : Integrator
  Saturation1 : Saturate  UpperLimit=1.72  LowerLimit=-1.72
  Sum : Sum  Inputs=|+-
  Sum1 : Sum  Inputs=-+|
  Transfer Fcn : TransferFcn  Numerator=[1/R]  Denominator=[L/R 1]
  Out1: Iд : Outport  VectorParamsAs1DForOutWhenUnconnected=off
  Out2: wд : Outport  Port=2  VectorParamsAs1DForOutWhenUnconnected=off
  wires:
  In1: Uд/1 -> Sum/1
  Transfer Fcn/1 -> Saturation1/1  "Iд"
  Sum/1 -> Transfer Fcn/1  "Uд - E"
  Integrator/1 -> Out2: wд/1, Gain2/1  "скорость"
  Gain2/1 -> Sum/2  "E"
  Gain1/1 -> Integrator/1  "ускорение"
  Gain/1 -> Sum1/2  "Mд"
  In2: Mвн/1 -> Sum1/1
  Sum1/1 -> Gain1/1
  Saturation1/1 -> Out1: Iд/1, Gain/1

== system six_rod_tensegrity_model_2021a/Control system/Motor2 ==
  In2: Mвн : Inport
  In1: Uд : Inport  Port=2
  Gain : Gain  Gain=km
  Gain1 : Gain  Gain=1/Jsum
  Gain2 : Gain  Gain=kw
  Integrator : Integrator
  Saturation1 : Saturate  UpperLimit=1.72  LowerLimit=-1.72
  Sum : Sum  Inputs=|+-
  Sum1 : Sum  Inputs=-+|
  Transfer Fcn : TransferFcn  Numerator=[1/R]  Denominator=[L/R 1]
  Out1: Iд : Outport  VectorParamsAs1DForOutWhenUnconnected=off
  Out2: wд : Outport  Port=2  VectorParamsAs1DForOutWhenUnconnected=off
  wires:
  In1: Uд/1 -> Sum/1
  Transfer Fcn/1 -> Saturation1/1  "Iд"
  Sum/1 -> Transfer Fcn/1  "Uд - E"
  Integrator/1 -> Out2: wд/1, Gain2/1  "скорость"
  Gain2/1 -> Sum/2  "E"
  Gain1/1 -> Integrator/1  "ускорение"
  Gain/1 -> Sum1/2  "Mд"
  In2: Mвн/1 -> Sum1/1
  Sum1/1 -> Gain1/1
  Saturation1/1 -> Out1: Iд/1, Gain/1

== system six_rod_tensegrity_model_2021a/Control system/Motor3 ==
  In2: Mвн : Inport
  In1: Uд : Inport  Port=2
  Gain : Gain  Gain=km
  Gain1 : Gain  Gain=1/Jsum
  Gain2 : Gain  Gain=kw
  Integrator : Integrator
  Saturation1 : Saturate  UpperLimit=1.72  LowerLimit=-1.72
  Sum : Sum  Inputs=|+-
  Sum1 : Sum  Inputs=-+|
  Transfer Fcn : TransferFcn  Numerator=[1/R]  Denominator=[L/R 1]
  Out1: Iд : Outport  VectorParamsAs1DForOutWhenUnconnected=off
  Out2: wд : Outport  Port=2  VectorParamsAs1DForOutWhenUnconnected=off
  wires:
  In1: Uд/1 -> Sum/1
  Transfer Fcn/1 -> Saturation1/1  "Iд"
  Sum/1 -> Transfer Fcn/1  "Uд - E"
  Integrator/1 -> Out2: wд/1, Gain2/1  "скорость"
  Gain2/1 -> Sum/2  "E"
  Gain1/1 -> Integrator/1  "ускорение"
  Gain/1 -> Sum1/2  "Mд"
  In2: Mвн/1 -> Sum1/1
  Sum1/1 -> Gain1/1
  Saturation1/1 -> Out1: Iд/1, Gain/1

== system six_rod_tensegrity_model_2021a/Control system/Motor4 ==
  In2: Mвн : Inport
  In1: Uд : Inport  Port=2
  Gain : Gain  Gain=km
  Gain1 : Gain  Gain=1/Jsum
  Gain2 : Gain  Gain=kw
  Integrator : Integrator
  Saturation1 : Saturate  UpperLimit=1.72  LowerLimit=-1.72
  Sum : Sum  Inputs=|+-
  Sum1 : Sum  Inputs=-+|
  Transfer Fcn : TransferFcn  Numerator=[1/R]  Denominator=[L/R 1]
  Out1: Iд : Outport  VectorParamsAs1DForOutWhenUnconnected=off
  Out2: wд : Outport  Port=2  VectorParamsAs1DForOutWhenUnconnected=off
  wires:
  In1: Uд/1 -> Sum/1
  Transfer Fcn/1 -> Saturation1/1  "Iд"
  Sum/1 -> Transfer Fcn/1  "Uд - E"
  Integrator/1 -> Out2: wд/1, Gain2/1  "скорость"
  Gain2/1 -> Sum/2  "E"
  Gain1/1 -> Integrator/1  "ускорение"
  Gain/1 -> Sum1/2  "Mд"
  In2: Mвн/1 -> Sum1/1
  Sum1/1 -> Gain1/1
  Saturation1/1 -> Out1: Iд/1, Gain/1

== system six_rod_tensegrity_model_2021a/Control system/Motor5 ==
  In2: Mвн : Inport
  In1: Uд : Inport  Port=2
  Gain : Gain  Gain=km
  Gain1 : Gain  Gain=1/Jsum
  Gain2 : Gain  Gain=kw
  Integrator : Integrator
  Saturation1 : Saturate  UpperLimit=1.72  LowerLimit=-1.72
  Sum : Sum  Inputs=|+-
  Sum1 : Sum  Inputs=-+|
  Transfer Fcn : TransferFcn  Numerator=[1/R]  Denominator=[L/R 1]
  Out1: Iд : Outport  VectorParamsAs1DForOutWhenUnconnected=off
  Out2: wд : Outport  Port=2  VectorParamsAs1DForOutWhenUnconnected=off
  wires:
  In1: Uд/1 -> Sum/1
  Transfer Fcn/1 -> Saturation1/1  "Iд"
  Sum/1 -> Transfer Fcn/1  "Uд - E"
  Integrator/1 -> Out2: wд/1, Gain2/1  "скорость"
  Gain2/1 -> Sum/2  "E"
  Gain1/1 -> Integrator/1  "ускорение"
  Gain/1 -> Sum1/2  "Mд"
  In2: Mвн/1 -> Sum1/1
  Sum1/1 -> Gain1/1
  Saturation1/1 -> Out1: Iд/1, Gain/1

== system six_rod_tensegrity_model_2021a/Control system/Внешний момент ==
  Demux : Demux  Tag=STV Demux  Outputs=1
      settings: DisplayOption=none
  FromWs : FromWorkspace  Tag=STV FromWs  VariableName=tuvar
      SigBuilderData=|
      | common.afterFinalStr = 'Extrapolate'
      | common.sampleTime = 0
      | dataSet.timeRange = [0 10]
      | dataSet.name = 'Group 1'
      | sbobj.Groups.Name = 'Group 1'
      | sbobj.Groups.Signals.Name = 'Signal 1'
      | sbobj.Groups.Signals.XData = [0 2 3 5 10]
      | sbobj.Groups.Signals.YData = [0.129 0.08 0.08 0.129 0.129]
  Signal 1 : Outport  Tag=STV Outport  VectorParamsAs1DForOutWhenUnconnected=off
  wires:
  FromWs/1 -> Demux/1
  Demux/1 -> Signal 1/1

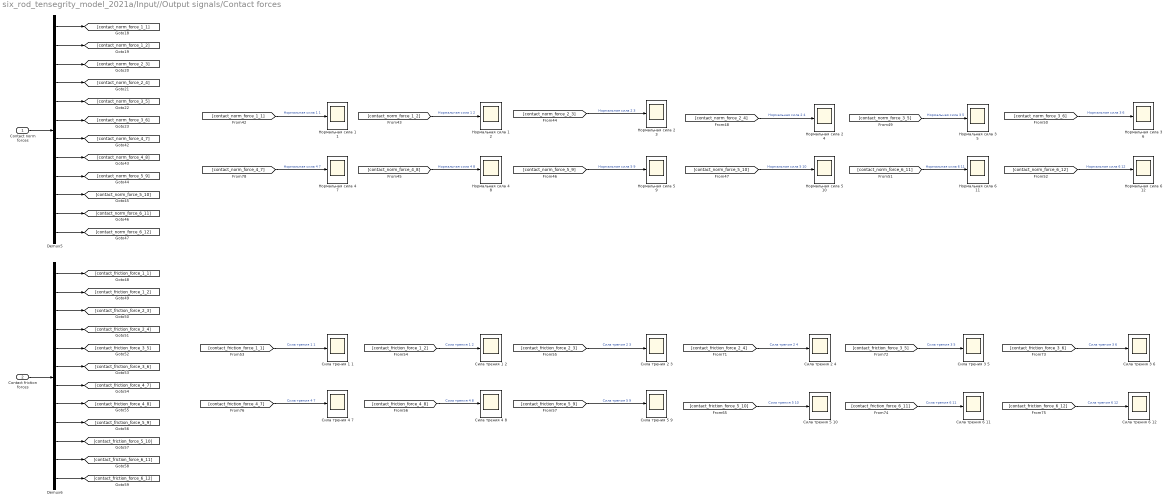
== system six_rod_tensegrity_model_2021a/Input//Output signals/Contact forces ==
  Contact norm forces : Inport
  Contact friction forces : Inport  Port=2
  Demux5 : Demux  Outputs=12
  Demux6 : Demux  Outputs=12
  Нормальная сила 1 1 : Scope
  Нормальная сила 1 2 : Scope
  Нормальная сила 2 3 : Scope
  Нормальная сила 2 4 : Scope
  Нормальная сила 3 5 : Scope
  Нормальная сила 3 6 : Scope
  Нормальная сила 4 7 : Scope
  Нормальная сила 4 8 : Scope
  Нормальная сила 5 10 : Scope
  Нормальная сила 5 9 : Scope
  Нормальная сила 6 11 : Scope
  Нормальная сила 6 12 : Scope
  Сила трения 1 1 : Scope
  Сила трения 1 2 : Scope
  Сила трения 2 3 : Scope
  Сила трения 2 4 : Scope
  Сила трения 3 5 : Scope
  Сила трения 3 6 : Scope
  Сила трения 4 7 : Scope
  Сила трения 4 8 : Scope
  Сила трения 5 10 : Scope
  Сила трения 5 9 : Scope
  Сила трения 6 11 : Scope
  Сила трения 6 12 : Scope
  wires:
  Demux5/5 -> [contact_norm_force_3_5]
  Demux5/11 -> [contact_norm_force_6_11]
  [contact_norm_force_1_1] -> Нормальная сила 1 1/1  "Нормальная сила 1 1"
  [contact_norm_force_2_3] -> Нормальная сила 2 3/1  "Нормальная сила 2 3"
  Demux6/11 -> [contact_friction_force_6_11]
  [contact_friction_force_5_9] -> Сила трения 5 9/1  "Сила трения 5 9"
  [contact_friction_force_6_12] -> Сила трения 6 12/1  "Сила трения 6 12"
  [contact_friction_force_5_10] -> Сила трения 5 10/1  "Сила трения 5 10"
  Demux5/6 -> [contact_norm_force_3_6]
  Demux5/2 -> [contact_norm_force_1_2]
  [contact_norm_force_4_7] -> Нормальная сила 4 7/1  "Нормальная сила 4 7"
  Demux5/4 -> [contact_norm_force_2_4]
  Demux5/8 -> [contact_norm_force_4_8]
  Demux5/7 -> [contact_norm_force_4_7]
  [contact_norm_force_3_6] -> Нормальная сила 3 6/1  "Нормальная сила 3 6"
  Demux5/3 -> [contact_norm_force_2_3]
  Demux5/12 -> [contact_norm_force_6_12]
  Demux6/1 -> [contact_friction_force_1_1]
  [contact_norm_force_2_4] -> Нормальная сила 2 4/1  "Нормальная сила 2 4"
  Demux6/4 -> [contact_friction_force_2_4]
  Demux6/5 -> [contact_friction_force_3_5]
  [contact_norm_force_4_8] -> Нормальная сила 4 8/1  "Нормальная сила 4 8"
  Demux6/8 -> [contact_friction_force_4_8]
  Demux6/2 -> [contact_friction_force_1_2]
  Contact friction forces/1 -> Demux6/1
  Demux6/3 -> [contact_friction_force_2_3]
  Demux5/10 -> [contact_norm_force_5_10]
  [contact_norm_force_6_11] -> Нормальная сила 6 11/1  "Нормальная сила 6 11"
  Demux6/7 -> [contact_friction_force_4_7]
  Demux6/12 -> [contact_friction_force_6_12]
  Demux6/10 -> [contact_friction_force_5_10]
  [contact_friction_force_4_8] -> Сила трения 4 8/1  "Сила трения 4 8"
  Demux6/9 -> [contact_friction_force_5_9]
  [contact_norm_force_5_10] -> Нормальная сила 5 10/1  "Нормальная сила 5 10"
  Demux5/1 -> [contact_norm_force_1_1]
  Demux6/6 -> [contact_friction_force_3_6]
  [contact_friction_force_2_4] -> Сила трения 2 4/1  "Сила трения 2 4"
  [contact_friction_force_4_7] -> Сила трения 4 7/1  "Сила трения 4 7"
  [contact_norm_force_6_12] -> Нормальная сила 6 12/1  "Нормальная сила 6 12"
  [contact_friction_force_2_3] -> Сила трения 2 3/1  "Сила трения 2 3"
  Contact norm forces/1 -> Demux5/1
  [contact_friction_force_1_1] -> Сила трения 1 1/1  "Сила трения 1 1"
  [contact_friction_force_3_5] -> Сила трения 3 5/1  "Сила трения 3 5"
  [contact_friction_force_6_11] -> Сила трения 6 11/1  "Сила трения 6 11"
  [contact_friction_force_1_2] -> Сила трения 1 2/1  "Сила трения 1 2"
  [contact_norm_force_1_2] -> Нормальная сила 1 2/1  "Нормальная сила 1 2"
  [contact_norm_force_5_9] -> Нормальная сила 5 9/1  "Нормальная сила 5 9"
  [contact_norm_force_3_5] -> Нормальная сила 3 5/1  "Нормальная сила 3 5"
  [contact_friction_force_3_6] -> Сила трения 3 6/1  "Сила трения 3 6"
  Demux5/9 -> [contact_norm_force_5_9]

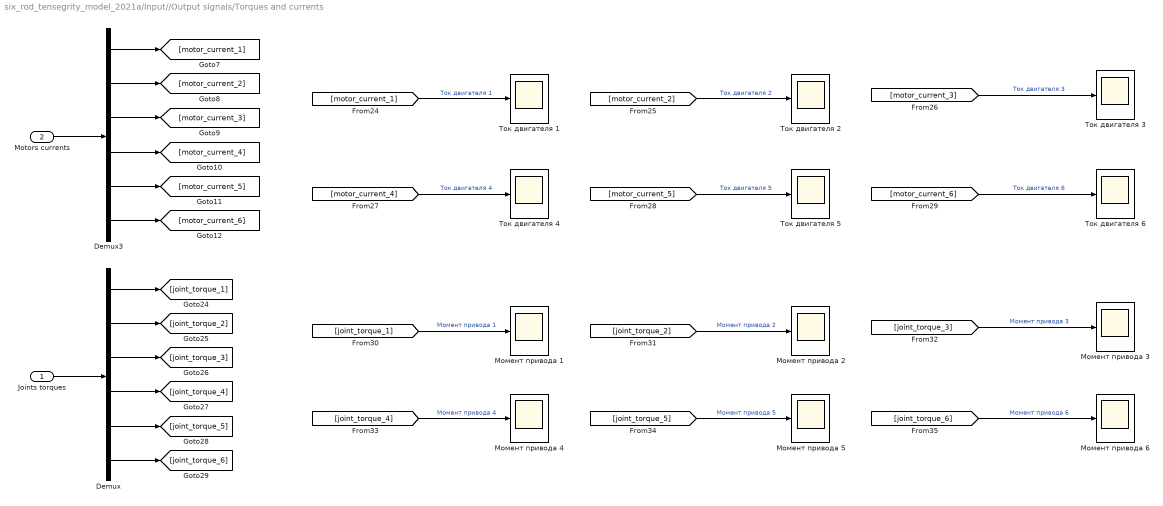
== system six_rod_tensegrity_model_2021a/Input//Output signals/Torques and currents ==
  Joints torques : Inport
  Motors currents : Inport  Port=2
  Demux : Demux  Outputs=6
  Demux3 : Demux  Outputs=6
  Момент привода {1..6} (6 alike) : Scope
  Ток двигателя {1..6} (6 alike) : Scope
  wires:
  [motor_current_5] -> Ток двигателя 5/1  "Ток двигателя 5"
  Demux3/6 -> [motor_current_6]
  [joint_torque_4] -> Момент привода 4/1  "Момент привода 4"
  Demux3/3 -> [motor_current_3]
  [joint_torque_1] -> Момент привода 1/1  "Момент привода 1"
  Demux3/5 -> [motor_current_5]
  Demux/6 -> [joint_torque_6]
  Demux3/1 -> [motor_current_1]
  Demux3/2 -> [motor_current_2]
  Motors currents/1 -> Demux3/1
  Demux3/4 -> [motor_current_4]
  [joint_torque_5] -> Момент привода 5/1  "Момент привода 5"
  [joint_torque_2] -> Момент привода 2/1  "Момент привода 2"
  [joint_torque_6] -> Момент привода 6/1  "Момент привода 6"
  Demux/5 -> [joint_torque_5]
  [joint_torque_3] -> Момент привода 3/1  "Момент привода 3"
  [motor_current_3] -> Ток двигателя 3/1  "Ток двигателя 3"
  [motor_current_4] -> Ток двигателя 4/1  "Ток двигателя 4"
  [motor_current_6] -> Ток двигателя 6/1  "Ток двигателя 6"
  Demux/2 -> [joint_torque_2]
  Demux/1 -> [joint_torque_1]
  Demux/3 -> [joint_torque_3]
  Demux/4 -> [joint_torque_4]
  Joints torques/1 -> Demux/1
  [motor_current_1] -> Ток двигателя 1/1  "Ток двигателя 1"
  [motor_current_2] -> Ток двигателя 2/1  "Ток двигателя 2"

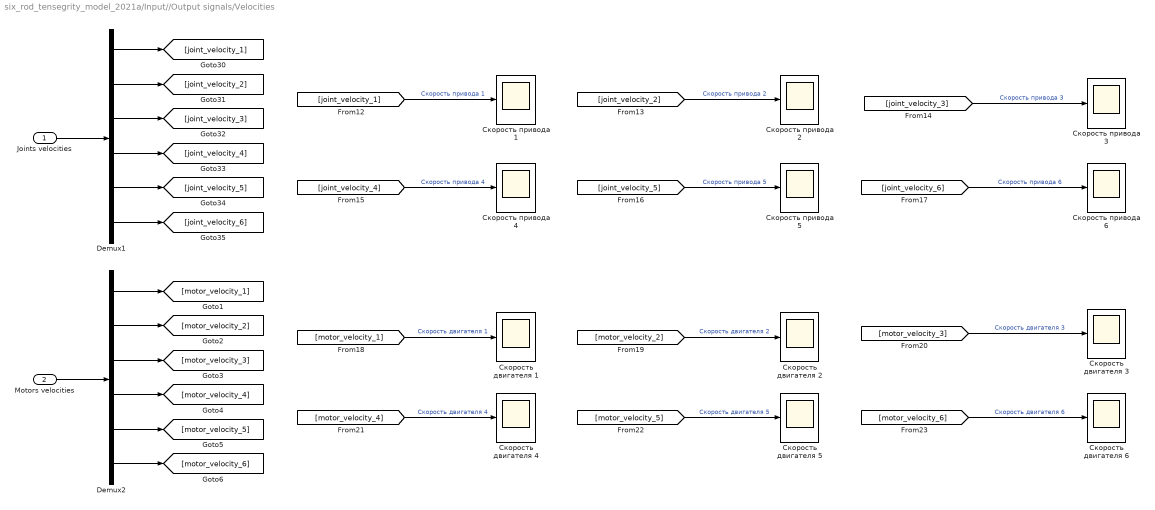
== system six_rod_tensegrity_model_2021a/Input//Output signals/Velocities ==
  Joints velocities : Inport
  Motors velocities : Inport  Port=2
  Demux1 : Demux  Outputs=6
  Demux2 : Demux  Outputs=6
  Скорость двигателя {1..6} (6 alike) : Scope
  Скорость привода {1..6} (6 alike) : Scope
  wires:
  Motors velocities/1 -> Demux2/1
  Demux1/5 -> [joint_velocity_5]
  Demux1/2 -> [joint_velocity_2]
  Demux1/1 -> [joint_velocity_1]
  [joint_velocity_1] -> Скорость привода 1/1  "Скорость привода 1"
  [joint_velocity_2] -> Скорость привода 2/1  "Скорость привода 2"
  [joint_velocity_3] -> Скорость привода 3/1  "Скорость привода 3"
  Demux1/4 -> [joint_velocity_4]
  [joint_velocity_5] -> Скорость привода 5/1  "Скорость привода 5"
  [motor_velocity_1] -> Скорость двигателя 1/1  "Скорость двигателя 1"
  Demux1/3 -> [joint_velocity_3]
  Demux2/2 -> [motor_velocity_2]
  [motor_velocity_2] -> Скорость двигателя 2/1  "Скорость двигателя 2"
  Demux1/6 -> [joint_velocity_6]
  Joints velocities/1 -> Demux1/1
  [joint_velocity_4] -> Скорость привода 4/1  "Скорость привода 4"
  Demux2/5 -> [motor_velocity_5]
  Demux2/4 -> [motor_velocity_4]
  Demux2/3 -> [motor_velocity_3]
  Demux2/6 -> [motor_velocity_6]
  [motor_velocity_6] -> Скорость двигателя 6/1  "Скорость двигателя 6"
  Demux2/1 -> [motor_velocity_1]
  [motor_velocity_3] -> Скорость двигателя 3/1  "Скорость двигателя 3"
  [motor_velocity_5] -> Скорость двигателя 5/1  "Скорость двигателя 5"
  [motor_velocity_4] -> Скорость двигателя 4/1  "Скорость двигателя 4"
  [joint_velocity_6] -> Скорость привода 6/1  "Скорость привода 6"
